simulink model "sampleModel35"  (R2021b)
settings: Solver=VariableStepAuto  StartTime=0.0  StopTime=10.0  RelTol=1e-3
libraries: simulink x2
settings Model: Creator=user  LastModifiedBy=user

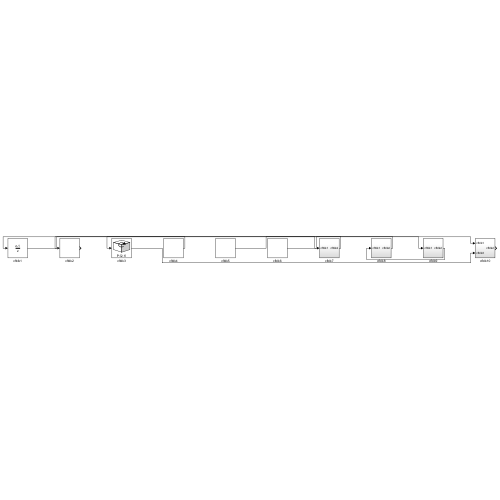
[thumbnail: Simulink's stored preview of the top-level diagram]
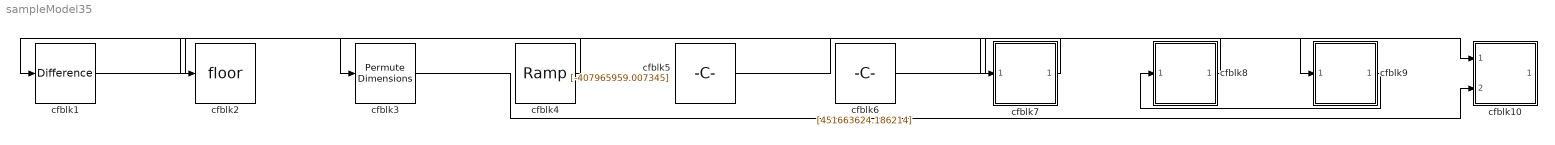
== system sampleModel35 ==
  cfblk1 : simulink/Discrete/Difference  ICPrevInput=0.0  OutMin=[]  OutMax=[]  OutDataTypeStr=Inherit: Inherit via back propagation  OutDataType=fixdt(1, 16)  OutScaling=2^-10  DoSatur=off
  cfblk10 : Subsystem
  cfblk2 : Rounding
  cfblk3 : PermuteDimensions
  cfblk4 : simulink/Sources/Ramp  slope=[6518.682181]  start=[45.879952]  InitialOutput=[-465293.955274]
  cfblk5 : Constant  Value=[-407965959.007345]  SampleTime=1
  cfblk6 : Constant  Value=[451663624.186214]  SampleTime=1
  cfblk7 : Subsystem
  cfblk8 : Subsystem
  cfblk9 : Subsystem
  wires:
  cfblk6/1 -> cfblk10/1(cfblk1)
  cfblk1/1 -> cfblk7/1(cfblk1)
  cfblk9/1(cfblk2) -> cfblk8/1(cfblk1)
  cfblk3/1 -> cfblk10/2(cfblk3)
  cfblk8/1(cfblk2) -> cfblk3/1
  cfblk5/1 -> cfblk9/1(cfblk1)
  cfblk4/1 -> cfblk1/1
  cfblk7/1(cfblk2) -> cfblk2/1

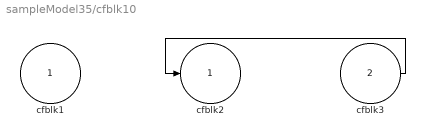
== system sampleModel35/cfblk10 ==
  cfblk1 : Inport
  cfblk3 : Inport  Port=2
  cfblk2 : Outport
  wires:
  cfblk3/1 -> cfblk2/1

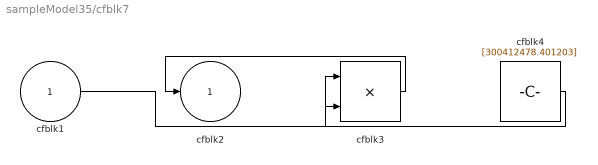
== system sampleModel35/cfblk7 ==
  cfblk1 : Inport
  cfblk3 : Product
  cfblk4 : Constant  Value=[300412478.401203]  SampleTime=1
  cfblk2 : Outport
  wires:
  cfblk3/1 -> cfblk2/1
  cfblk1/1 -> cfblk3/1
  cfblk4/1 -> cfblk3/2

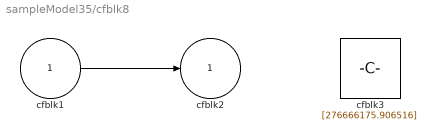
== system sampleModel35/cfblk8 ==
  cfblk1 : Inport
  cfblk3 : Constant  Value=[276666175.906516]  SampleTime=1
  cfblk2 : Outport
  wires:
  cfblk1/1 -> cfblk2/1

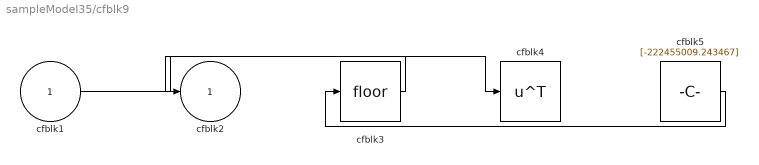
== system sampleModel35/cfblk9 ==
  cfblk1 : Inport
  cfblk3 : Rounding
  cfblk4 : Math  Operator=transpose  SaturateOnIntegerOverflow=on
  cfblk5 : Constant  Value=[-222455009.243467]  SampleTime=1
  cfblk2 : Outport
  wires:
  cfblk1/1 -> cfblk4/1
  cfblk5/1 -> cfblk3/1
  cfblk3/1 -> cfblk2/1
